simulink model "SyS_P1_Starset_Israel_Fonseca"  (R2019a)
settings: Solver=VariableStepAuto  StartTime=0.0  StopTime=10.0  RelTol=1e-3
settings Model: Creator=ifons  LastModifiedBy=ifons
settings DataIOCC: Refine=10

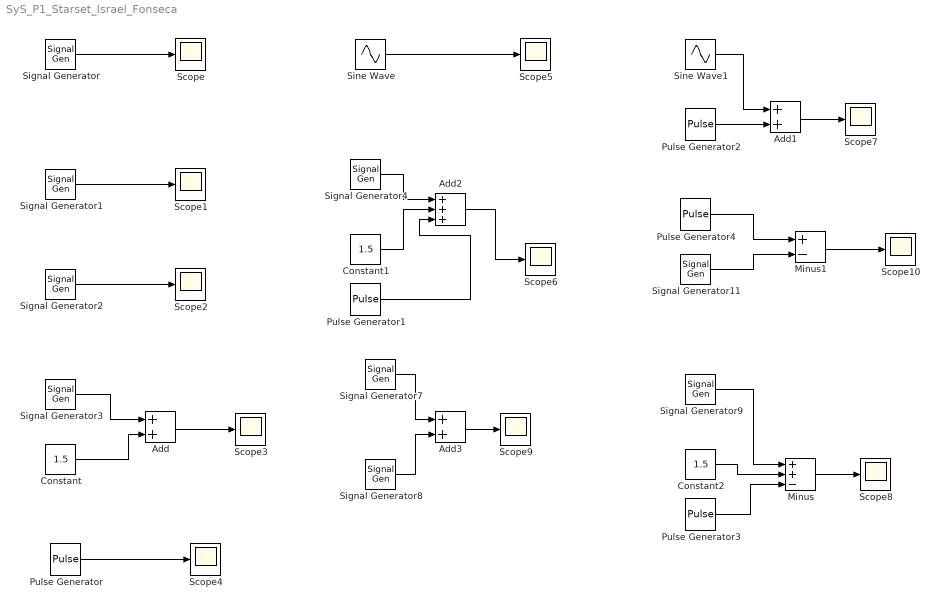
== system SyS_P1_Starset_Israel_Fonseca ==
  Add : Sum
  Add1 : Sum
  Add2 : Sum  Inputs=+++
  Add3 : Sum
  Constant : Constant  Value=1.5
  Constant1 : Constant  Value=1.5
  Constant2 : Constant  Value=1.5
  Minus : Sum  Inputs=++-
  Minus1 : Sum  Inputs=+-
  Pulse Generator{,1..4} (5 alike) : DiscretePulseGenerator  PulseType=Time based  Amplitude=5  Period=0.00002  PulseWidth=25
  Scope{,1..10} (11 alike) : Scope
  Signal Generator : SignalGenerator  Frequency=10
  Signal Generator1 : SignalGenerator  WaveForm=square  Frequency=10
  Signal Generator11 : SignalGenerator  Amplitude=4  Frequency=1000
  Signal Generator2 : SignalGenerator  Amplitude=4  Frequency=1000
  Signal Generator3 : SignalGenerator  WaveForm=sawtooth  Amplitude=1.5  Frequency=175
  Signal Generator4 : SignalGenerator  WaveForm=sawtooth  Amplitude=1.5  Frequency=175
  Signal Generator7 : SignalGenerator  WaveForm=square  Frequency=10
  Signal Generator8 : SignalGenerator  Amplitude=4  Frequency=1000
  Signal Generator9 : SignalGenerator  WaveForm=sawtooth  Amplitude=1.5  Frequency=175
  Sine Wave : Sin  Amplitude=5  Frequency=62831.853  Phase=-pi/4  SampleTime=0
  Sine Wave1 : Sin  Amplitude=5  Frequency=62831.853  Phase=-pi/4  SampleTime=0
  wires:
  Signal Generator/1 -> Scope/1
  Signal Generator1/1 -> Scope1/1
  Signal Generator2/1 -> Scope2/1
  Signal Generator3/1 -> Add/1
  Constant/1 -> Add/2
  Add/1 -> Scope3/1
  Pulse Generator/1 -> Scope4/1
  Constant1/1 -> Add2/2
  Add2/1 -> Scope6/1
  Signal Generator4/1 -> Add2/1
  Pulse Generator1/1 -> Add2/3
  Pulse Generator2/1 -> Add1/2
  Add1/1 -> Scope7/1
  Signal Generator7/1 -> Add3/1
  Signal Generator8/1 -> Add3/2
  Add3/1 -> Scope9/1
  Constant2/1 -> Minus/2
  Signal Generator9/1 -> Minus/1
  Pulse Generator3/1 -> Minus/3
  Minus/1 -> Scope8/1
  Minus1/1 -> Scope10/1
  Pulse Generator4/1 -> Minus1/1
  Signal Generator11/1 -> Minus1/2
  Sine Wave/1 -> Scope5/1
  Sine Wave1/1 -> Add1/1
